simulink model "DC_MOTOR_SIMULINK"  (R2022b)
settings: Solver=VariableStepAuto  StartTime=0.0  StopTime=10.0  RelTol=1e-3
values from neighbouring files (symbols this model uses):
  b = 3.5077E-6    (= 3.5077e-06)    [DC_MOTOR_Script.m]
  J = 3.2284E-6    (= 3.2284e-06)    [DC_MOTOR_Script.m]
  Kb = 0.0274    [DC_MOTOR_Script.m]
  Kt = 0.0274    [DC_MOTOR_Script.m]
  L = 2.75E-6    (= 2.75e-06)    [DC_MOTOR_Script.m]
  R = 4    [DC_MOTOR_Script.m]
  V = 1    [DC_MOTOR_Script.m]
undefined symbols (not defined in the file or in its folder): kd, ki, kp
settings Model: Creator=James  LastModifiedBy=James

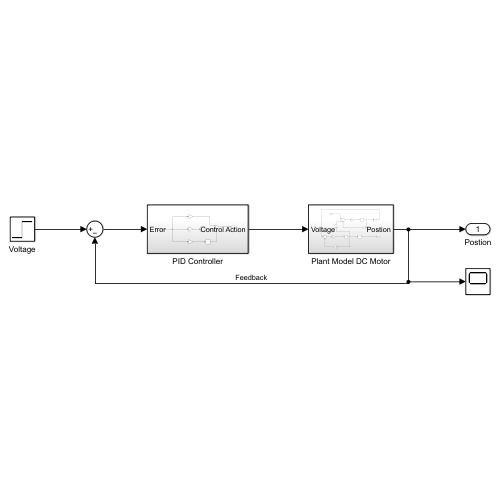
[thumbnail: Simulink's stored preview of the top-level diagram]
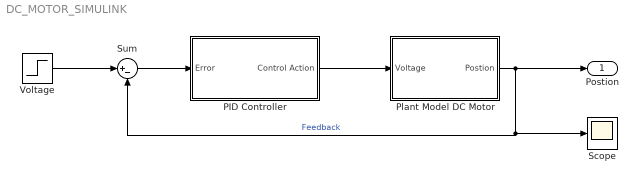
== system DC_MOTOR_SIMULINK ==
  PID Controller : Subsystem
  Plant Model DC Motor : Subsystem
  Scope : Scope
  Sum : Sum  Inputs=|+-
  Voltage : Step  After=V  SampleTime=0
  Postion : Outport
  wires:
  PID Controller/1(Control Action) -> Plant Model DC Motor/1(Voltage)
  Plant Model DC Motor/1(Postion) -> Scope/1, Sum/2, Postion/1  "Feedback"
  Voltage/1 -> Sum/1
  Sum/1 -> PID Controller/1(Error)

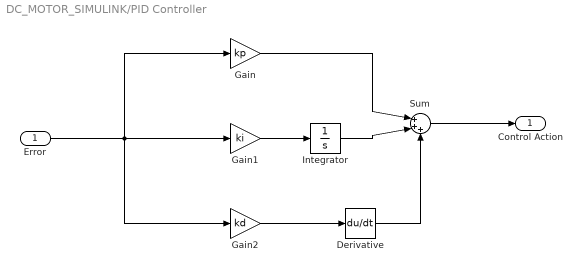
== system DC_MOTOR_SIMULINK/PID Controller ==
  Error : Inport
  Derivative : Derivative
  Gain : Gain  Gain=kp
  Gain1 : Gain  Gain=ki
  Gain2 : Gain  Gain=kd
  Integrator : Integrator
  Sum : Sum  Inputs=|+++
  Control Action : Outport
  wires:
  Derivative/1 -> Sum/3
  Error/1 -> Gain2/1, Gain/1, Gain1/1
  Sum/1 -> Control Action/1
  Gain/1 -> Sum/1
  Gain1/1 -> Integrator/1
  Integrator/1 -> Sum/2
  Gain2/1 -> Derivative/1

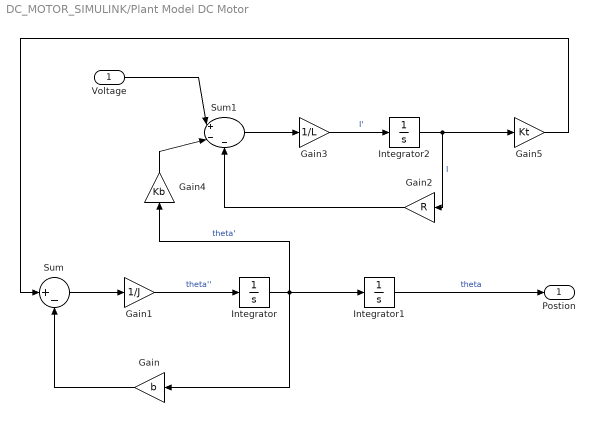
== system DC_MOTOR_SIMULINK/Plant Model DC Motor ==
  Voltage : Inport
  Gain : Gain  Gain=b
  Gain1 : Gain  Gain=1/J
  Gain2 : Gain  Gain=R
  Gain3 : Gain  Gain=1/L
  Gain4 : Gain  Gain=Kb
  Gain5 : Gain  Gain=Kt
  Integrator : Integrator
  Integrator1 : Integrator
  Integrator2 : Integrator
  Sum : Sum  Inputs=|+-
  Sum1 : Sum  Inputs=|+--
  Postion : Outport
  wires:
  Integrator2/1 -> Gain5/1, Gain2/1  "I"
  Sum1/1 -> Gain3/1
  Integrator/1 -> Gain4/1, Gain/1, Integrator1/1  "theta'"
  Sum/1 -> Gain1/1
  Gain/1 -> Sum/2
  Voltage/1 -> Sum1/1
  Gain1/1 -> Integrator/1  "theta''"
  Gain4/1 -> Sum1/2
  Gain2/1 -> Sum1/3
  Gain3/1 -> Integrator2/1  "I'"
  Gain5/1 -> Sum/1
  Integrator1/1 -> Postion/1  "theta"
